simulink model "mysys"  (R2013a)
settings: Solver=ode45  StartTime=0.0  StopTime=10.0  RelTol=1e-3
libraries: simulink x2
settings Model: Creator=zhan  LastModifiedBy=zhihan
settings DataIOCC: FinalStateName=xF  SaveFinalState=on  SaveCompleteFinalSimState=on  SignalLoggingSaveFormat=ModelDataLogs
settings OptimizationCC: InlineParams=on  ExpressionDepthLimit=2147483647
settings DebuggingCC: FcnCallInpInsideContextMsg=UseLocalSettings
settings GRTTargetCC: CombineOutputUpdateFcns=off  GRTInterface=on

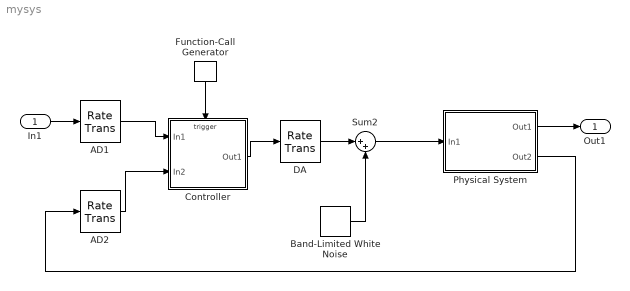
== system mysys ==
  In1 : Inport  SampleTime=0
  AD1 : RateTransition
  AD2 : RateTransition
  Band-Limited White Noise : simulink/Sources/Band-Limited White Noise  Cov=1e-4  Ts=0.1  seed=[23341]
  Controller : Subsystem
  DA : RateTransition
  Function-Call Generator : simulink/Ports & Subsystems/Function-Call Generator  sample_time=0.2  numberOfIterations=1
  Physical System : Subsystem
  Sum2 : Sum  Inputs=|++
  Out1 : Outport
  wires:
  In1/1 -> AD1/1
  Function-Call Generator/1 -> Controller/Trigger
  Controller/1(Out1) -> DA/1
  Sum2/1 -> Physical System/1(In1)
  Band-Limited White Noise/1 -> Sum2/2
  AD1/1 -> Controller/1(In1)
  AD2/1 -> Controller/2(In2)
  DA/1 -> Sum2/1
  Physical System/1(Out1) -> Out1/1
  Physical System/2(Out2) -> AD2/1

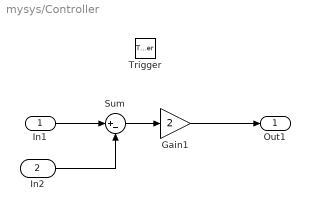
== system mysys/Controller ==
  In1 : Inport
  In2 : Inport  Port=2
  Trigger : TriggerPort  TriggerType=function-call
  Gain1 : Gain  Gain=2
  Sum : Sum  Inputs=|+-
  Out1 : Outport
  wires:
  Sum/1 -> Gain1/1
  In2/1 -> Sum/2
  Gain1/1 -> Out1/1
  In1/1 -> Sum/1

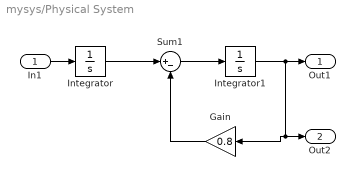
== system mysys/Physical System ==
  In1 : Inport
  Gain : Gain  Gain=0.8
  Integrator : Integrator
  Integrator1 : Integrator
  Sum1 : Sum  Inputs=|+-
  Out1 : Outport
  Out2 : Outport  Port=2
  wires:
  Integrator1/1 -> Gain/1, Out2/1, Out1/1
  Integrator/1 -> Sum1/1
  Sum1/1 -> Integrator1/1
  Gain/1 -> Sum1/2
  In1/1 -> Integrator/1
